simulink model "siso1"  (R2018a)
settings: Solver=VariableStepAuto  StartTime=0.0  StopTime=50.0  RelTol=1e-3
libraries: fuzblock x1
settings Model: Creator=root  LastModifiedBy=User
settings DebuggingCC: LibraryContextMissingDiagnostic=warning
settings SFSimCC: SimUseLocalCustomCode=on
settings RTWCC: RTWUseLocalCustomCode=on

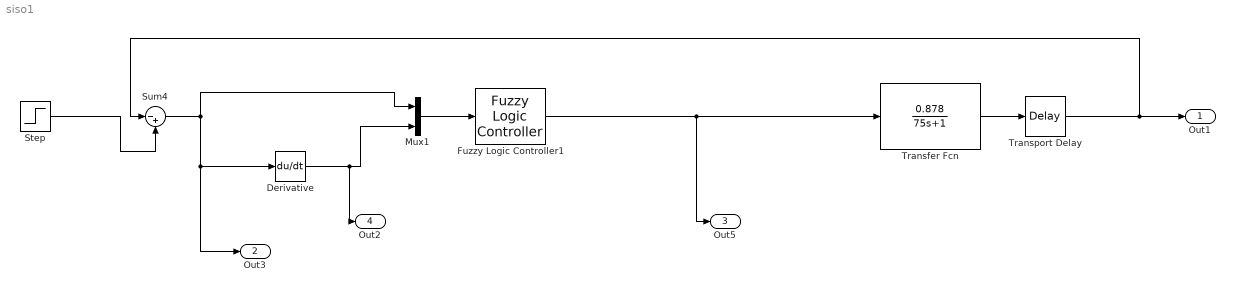
== system siso1 ==
  Derivative : Derivative
  Fuzzy Logic Controller1 : fuzblock/Fuzzy Logic  Controller  FIS=flc1  OutputSampleNumber=101  DataType=double  FuzzifiedInputs=off  RuleFiringStrengths=off  RuleOutputs=off  AggregatedOutputs=off  SimulateUsing=Interpreted execution  OutOfRangeInputValueMessage=warning  NoRuleFiredMessage=warning  EmptyOutputFuzzySetMessage=warning
  Mux1 : Mux  Inputs=2
  Step : Step  SampleTime=0
  Sum4 : Sum  Inputs=|-+
  Transfer Fcn : TransferFcn  Numerator=[0.878]  Denominator=[75 1]
  Transport Delay : TransportDelay
  Out1 : Outport  SignalName=y1
  Out3 : Outport  Port=2  SignalName=Erro1
  Out5 : Outport  Port=3  SignalName=Control1
  Out2 : Outport  Port=4  SignalName=Derivada_erro1
  wires:
  Transfer Fcn/1 -> Transport Delay/1
  Transport Delay/1 -> Sum4/1, Out1/1
  Step/1 -> Sum4/2
  Sum4/1 -> Out3/1, Derivative/1, Mux1/1
  Fuzzy Logic Controller1/1 -> Out5/1, Transfer Fcn/1
  Mux1/1 -> Fuzzy Logic Controller1/1
  Derivative/1 -> Out2/1, Mux1/2
